simulink model "simulacao_manipulador_scara_Anne"  (R2022b)
settings: Solver=ode1  StartTime=0.0  StopTime=20  FixedStep=1e-4  RelTol=1e-3
values from neighbouring files (symbols this model uses):
  L1_num = 0.525    [testeSCARA.m]
  L2_num = 0.330    (= 0.33)    [testeSCARA.m]
  Lf_num = 0.07673    [testeSCARA.m]
undefined symbols (not defined in the file or in its folder): deltat, dq_ci, Kd, Kp, L0_num, PA_0, PB_0, PD_0, q_ci, Tpi_0, trajetLin1
settings Model: Creator=alefp  LastModifiedBy=rodrigo
settings OptimizationCC: DefaultParameterBehavior=Inlined  ReuseModelBlockBuffer=on  EnhancedBackFolding=on  PassReuseOutputArgsThreshold=0  OptimizeBlockOrder=speed  DifferentSizesBufferReuse=on  OptimizationCustomize=off
settings DebuggingCC: ReadBeforeWriteMsg=DisableAll  WriteAfterWriteMsg=DisableAll  WriteAfterReadMsg=DisableAll  MultiTaskDSMMsg=none  ParameterTunabilityLossMsg=error
settings ModelReferenceCC: UpdateModelReferenceTargets=IfOutOfDate
settings SFSimCC: SFSimEcho=off  MATLABDynamicMemAlloc=off
settings CodeAppCC: ForceParamTrailComments=on  OperatorAnnotations=on

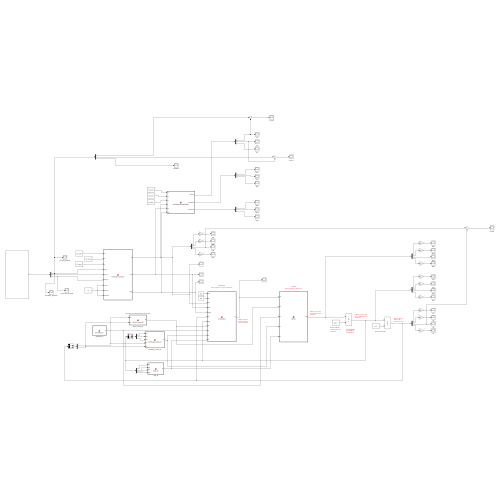
[thumbnail: Simulink's stored preview of the top-level diagram]
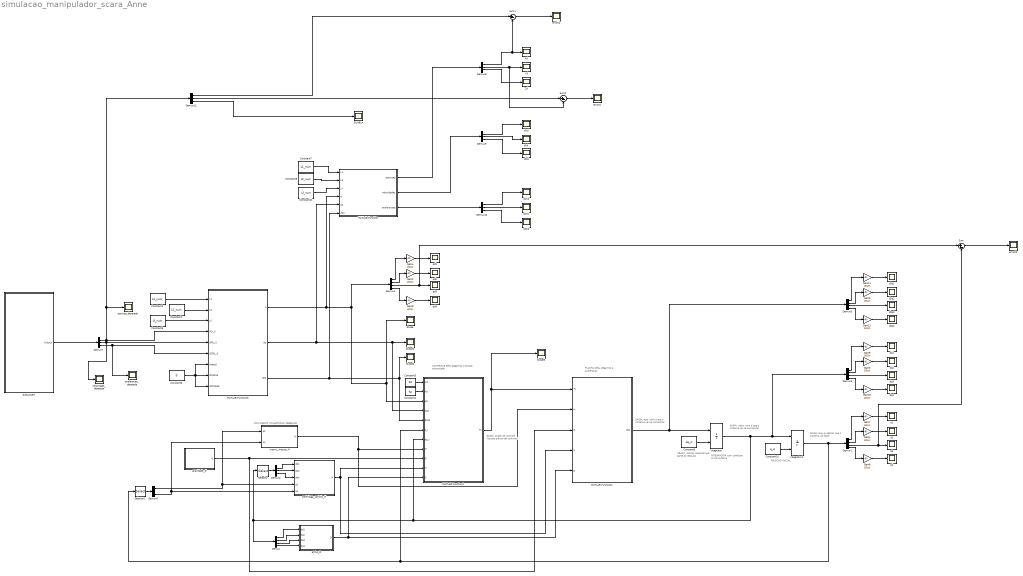
== system simulacao_manipulador_scara_Anne ==
  note: MOVIMENTO (TRAJETÓRIA) DESEJADO
  note: CONTROLE
      | Dele, pegamos o torque computado
  note: PLANTA
      | Dela, pegamos a aceleracao
  note: INTEGRADOR
      | com condicao inicial externa
  note: VELOC. INICIAL
      | Supondo que parte do repouso
  note: POSICAO INICIAL
  note: SAIDA: ang. ou desloc que o sistema vai fazer
  note: SAIDA: veloc. com a que o sistema vai se comportar
  note: SAIDA: acel. com a que o sistema vai se comportar
  note: SAIDA: acoes de controle (torque e forca de controle)
  BLABLA : Scope
  Constant1 : Constant  Value=L1_num
  Constant10 : Constant  Value=q_ci
  Constant11 : Constant  Value=Lf_num
  Constant2 : Constant  Value=L2_num
  Constant3 : Constant  Value=Kd
  Constant4 : Constant  Value=Kp
  Constant5 : Constant  Value=Lf_num
  Constant6 : Constant  Value=0
  Constant7 : Constant  Value=L1_num
  Constant8 : Constant  Value=L2_num
  Constant9 : Constant  Value=dq_ci
  Demux{,1,3..5} (5 alike) : Demux
  Demux{2,7..11} (6 alike) : Demux  Outputs=3
  Demux6 : Demux  Outputs=2
  Gain{1..12} (12 alike) : Gain  Gain=180/pi
  Integrator : Integrator  InitialConditionSource=external
  Integrator1 : Integrator  InitialConditionSource=external
  MATLAB Function : MATLAB Function  TreatAsAtomicUnit=on
  MATLAB Function1 : MATLAB Function  TreatAsAtomicUnit=on
  MATLAB Function2 : MATLAB Function  TreatAsAtomicUnit=on
  MATLAB Function3 : MATLAB Function  TreatAsAtomicUnit=on
  Scope{,1..3} (4 alike) : Scope
  Selector : Selector  InputPortWidth=4  IndexOptions=Index vector (dialog)  Indices=[1, 2, 4]  OutputSizes=1
  Selector1 : Selector  InputPortWidth=4  IndexOptions=Index vector (dialog)  Indices=[2, 4]  OutputSizes=1
  Subsystem : Subsystem
  Sum : Sum  Inputs=|+-
  Sum1 : Sum  Inputs=|+-
  Sum2 : Sum  Inputs=|+-
  Xd : Scope
  Yd : Scope
  Zd : Scope
  aceleracao_desejada : Scope
  atrito_D : MATLAB Function  TreatAsAtomicUnit=on
  centrifuga_coriolis_H : MATLAB Function  TreatAsAtomicUnit=on
  d2Xd : Scope
  d2Yd : Scope
  d2Zd : Scope
  d2q{1..4} (4 alike) : Scope
  dXd : Scope
  dYd : Scope
  dZd : Scope
  dq{1..4} (4 alike) : Scope
  erroQ3 : Scope
  erroXd : Scope
  erroYd : Scope
  gravidade_G : MATLAB Function  TreatAsAtomicUnit=on
  matriz_massa_M : MATLAB Function  TreatAsAtomicUnit=on
  posicao_desejada : Scope
  q{1..4} (4 alike) : Scope
  qd{1..4} (4 alike) : Scope
  velocidade_desejada : Scope
  wires:
  MATLAB Function3/2(dq) -> MATLAB Function/5(dq), MATLAB Function1/4(dqd), Scope1/1
  MATLAB Function3/3(d2q) -> MATLAB Function/6(d2q), MATLAB Function1/5(d2qd), Scope2/1
  MATLAB Function3/1(q) -> MATLAB Function/4(q), Scope/1, MATLAB Function1/3(qd), Demux4/1
  MATLAB Function1/1(Tc) -> Scope3/1, MATLAB Function2/1(Tc)
  Constant9/1 -> Integrator/2
  Constant10/1 -> Integrator1/2
  Demux4/1 -> Gain4/1
  Gain4/1 -> qd1/1
  matriz_massa_M/1(M) -> MATLAB Function2/2(M), MATLAB Function1/8(M)
  gravidade_G/1(G) -> MATLAB Function2/3(G), MATLAB Function1/9(G)
  centrifuga_coriolis_H/1(H) -> MATLAB Function1/10(H), MATLAB Function2/4(H)
  atrito_D/1(D) -> MATLAB Function1/11(D), MATLAB Function2/5(D)
  Gain2/1 -> qd2/1
  Demux4/2 -> Gain2/1
  Gain6/1 -> qd4/1
  Demux4/4 -> Gain6/1
  Demux/1 -> atrito_D/1(dq1)
  Demux/2 -> atrito_D/2(dq2)
  Demux/3 -> atrito_D/3(dq3)
  Demux/4 -> atrito_D/4(dq4)
  Demux2/2 -> centrifuga_coriolis_H/2(dq2)
  Demux2/1 -> centrifuga_coriolis_H/1(dq1)
  Selector/1 -> Demux2/1
  Demux6/1 -> matriz_massa_M/1(q2), centrifuga_coriolis_H/4(q2)
  Selector1/1 -> Demux6/1
  Demux1/4 -> Gain8/1
  Demux1/3 -> Sum/2, q3/1
  Demux1/1 -> Gain7/1
  Demux1/2 -> Gain1/1
  Integrator1/1 -> MATLAB Function1/6(q_r), Selector1/1, Demux1/1
  Gain1/1 -> q2/1
  Gain8/1 -> q4/1
  Gain7/1 -> q1/1
  Demux3/4 -> Gain10/1
  Demux3/3 -> dq3/1
  Demux3/1 -> Gain9/1
  Demux3/2 -> Gain3/1
  Integrator/1 -> Demux3/1, Integrator1/1, Selector/1, Demux/1, MATLAB Function1/7(dq_r)
  Gain3/1 -> dq2/1
  Gain10/1 -> dq4/1
  Gain9/1 -> dq1/1
  Demux5/4 -> Gain12/1
  Demux5/3 -> d2q3/1
  Demux5/1 -> Gain11/1
  Demux5/2 -> Gain5/1
  MATLAB Function2/1(d2q) -> Demux5/1, Integrator/1
  Gain5/1 -> d2q2/1
  Gain12/1 -> d2q4/1
  Gain11/1 -> d2q1/1
  Constant3/1 -> MATLAB Function1/1(Kd)
  Constant4/1 -> MATLAB Function1/2(Kp)
  Demux6/2 -> centrifuga_coriolis_H/5(q4), matriz_massa_M/2(q4)
  Constant1/1 -> MATLAB Function3/1(L1)
  Constant2/1 -> MATLAB Function3/2(L2)
  Constant5/1 -> MATLAB Function3/3(Lf)
  Constant6/1 -> MATLAB Function3/9(d2theta5), MATLAB Function3/7(theta5), MATLAB Function3/8(dtheta5)
  Demux7/2 -> velocidade_desejada/1, MATLAB Function3/5(dPQ_0)
  Demux7/3 -> MATLAB Function3/6(d2PQ_0), aceleracao_desejada/1
  Demux7/1 -> Demux11/1, posicao_desejada/1, MATLAB Function3/4(PQ_0)
  Subsystem/1(Output) -> Demux7/1
  Demux2/3 -> centrifuga_coriolis_H/3(dq4)
  Sum/1 -> erroQ3/1
  Constant7/1 -> MATLAB Function/1(L1)
  Constant8/1 -> MATLAB Function/2(L2)
  Constant11/1 -> MATLAB Function/3(Lf)
  Sum1/1 -> erroXd/1
  Demux4/3 -> Sum/1, qd3/1
  MATLAB Function/3(aceleracoes) -> Demux10/1
  MATLAB Function/2(velocidades) -> Demux9/1
  MATLAB Function/1(posicoes) -> Demux8/1
  Demux8/3 -> Zd/1
  Demux8/2 -> Sum2/2, Yd/1
  Demux8/1 -> Sum1/2, Xd/1
  Demux9/3 -> dZd/1
  Demux9/2 -> dYd/1
  Demux9/1 -> dXd/1
  Demux10/3 -> d2Zd/1
  Demux10/2 -> d2Yd/1
  Demux10/1 -> d2Xd/1
  Demux11/1 -> Sum1/1
  Demux11/2 -> Sum2/1
  Sum2/1 -> erroYd/1
  Demux11/3 -> BLABLA/1

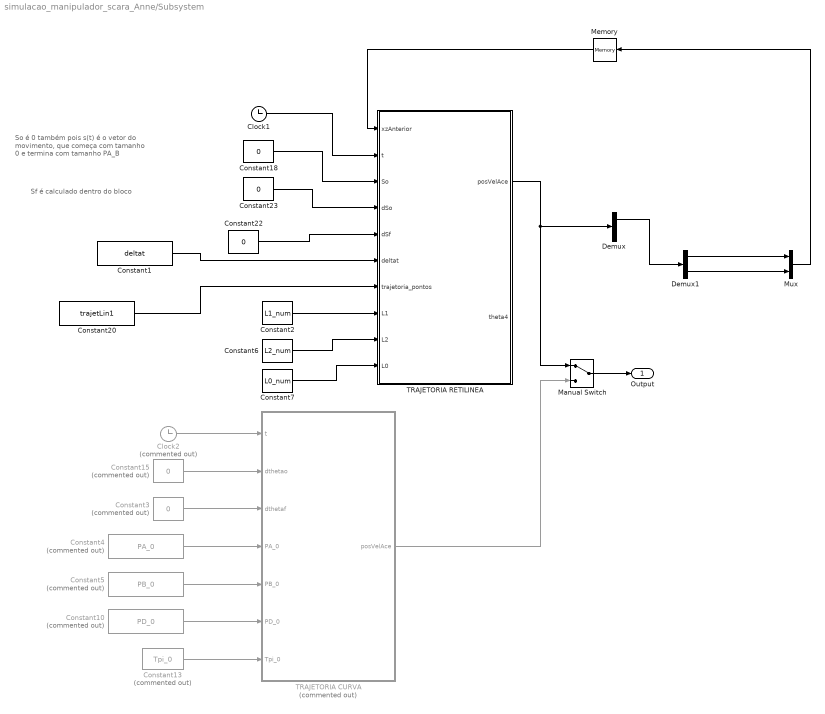
== system simulacao_manipulador_scara_Anne/Subsystem ==
  note: Sf é calculado dentro do bloco
  note: So é 0 também pois s(t) é o vetor do movimento, que começa com tamanho 0 e termina com tamanho PA_B
  Clock1 : Clock
  Clock2 : Clock  Commented=on
  Constant1 : Constant  Value=deltat
  Constant10 : Constant  Commented=on  Value=PD_0
  Constant13 : Constant  Commented=on  Value=Tpi_0
  Constant15 : Constant  Commented=on  Value=0
  Constant18 : Constant  Value=0
  Constant2 : Constant  Value=L1_num
  Constant20 : Constant  Value=trajetLin1
  Constant22 : Constant  Value=0
  Constant23 : Constant  Value=0
  Constant3 : Constant  Commented=on  Value=0
  Constant4 : Constant  Commented=on  Value=PA_0
  Constant5 : Constant  Commented=on  Value=PB_0
  Constant6 : Constant  Value=L2_num
  Constant7 : Constant  Value=L0_num
  Demux : Demux  Outputs=3
  Demux1 : Demux  Outputs=3
  Manual Switch : ManualSwitch
  Memory : Memory
  Mux : Mux  Inputs=2
  TRAJETORIA CURVA : MATLAB Function  Commented=on  TreatAsAtomicUnit=on
  TRAJETORIA RETILINEA : MATLAB Function  TreatAsAtomicUnit=on
  Output : Outport
  wires:
  Constant4/1 -> TRAJETORIA CURVA/4(PA_0)
  Constant3/1 -> TRAJETORIA CURVA/3(dthetaf)
  Clock2/1 -> TRAJETORIA CURVA/1(t)
  Constant15/1 -> TRAJETORIA CURVA/2(dthetao)
  Constant5/1 -> TRAJETORIA CURVA/5(PB_0)
  Constant10/1 -> TRAJETORIA CURVA/6(PD_0)
  Manual Switch/1 -> Output/1
  TRAJETORIA CURVA/1(posVelAce) -> Manual Switch/2
  Constant13/1 -> TRAJETORIA CURVA/7(Tpi_0)
  Constant22/1 -> TRAJETORIA RETILINEA/5(dSf)
  Clock1/1 -> TRAJETORIA RETILINEA/2(t)
  Constant18/1 -> TRAJETORIA RETILINEA/3(So)
  Constant23/1 -> TRAJETORIA RETILINEA/4(dSo)
  Constant1/1 -> TRAJETORIA RETILINEA/6(deltat)
  TRAJETORIA RETILINEA/1(posVelAce) -> Demux/1, Manual Switch/1
  Mux/1 -> Memory/1
  Memory/1 -> TRAJETORIA RETILINEA/1(xzAnterior)
  Demux/1 -> Demux1/1
  Demux1/1 -> Mux/1
  Demux1/3 -> Mux/2
  Constant20/1 -> TRAJETORIA RETILINEA/7(trajetoria_pontos)
  Constant2/1 -> TRAJETORIA RETILINEA/8(L1)
  Constant6/1 -> TRAJETORIA RETILINEA/9(L2)
  Constant7/1 -> TRAJETORIA RETILINEA/10(L0)

== matlab function simulacao_manipulador_scara_Anne/atrito_D ==
  data: dq1 input; D output; dq2 input; dq3 input; dq4 input
function D = atrito_D(dq1,dq2,dq3,dq4)
%#codegen

%    This function was generated by the Symbolic Math Toolbox version 24.2.
%    25-Sep-2024 18:08:51

% dq1 = complex(dq1);  % if required to enforce complex operations
% dq2 = complex(dq2);  % if required to enforce complex operations
% dq3 = complex(dq3);  % if required to enforce complex operations
% dq4 = complex(dq4);  % if required to enforce complex operations
D = [dq1.*9.321584999999999e-3;dq2.*2.192184e-2;dq3.*1.74398e-4;dq4.*2.754e-4];
end

== matlab function simulacao_manipulador_scara_Anne/MATLAB Function3 ==
  data: L1 input; L2 input; q output; Lf input; PQ_0 input; dPQ_0 input; d2PQ_0 input; theta5 input; dq output; d2q output; dtheta5 input; d2theta5 input
function [q, dq, d2q]  = cinematica_inversa(L1, L2, Lf, PQ_0,dPQ_0, d2PQ_0, theta5, dtheta5, d2theta5)
    % theta5 é o angulo final da ferramenta, conseguido pela tarefa. Lembrando que q4 = theta5 - q1 - q2 
    % PQ_0: Vetor de posicoes desejadas
    % dPQ_0: Vetor de velocidades desejadas (linear e angular)
    % d2PQ_0: Vetor de acelerações desejadas
    
    x5 = PQ_0(1);
    y5 = PQ_0(2);
    z5 = PQ_0(3);
    
    %% Cálculo de q3 (componente prismática)
    % q3 é o deslocamento da junta prismática
    q3 = y5 + Lf;
    
    num = (x5^2 + z5^2 - L1^2 - L2^2);
    den = (2*L1*L2);

    % Truncando na 3ª casa decimal
    num = fix(num * 1000) / 1000;
    den = fix(den * 1000) / 1000;
    q2 = acos(num/den);
    if sao_valores_proximos(q2,0) || sao_valores_proximos(q2,pi) || sao_valores_proximos(q2,2*pi)
        q2 =+ 0.087; % acrescentando 5 graus
    end
    

    %% Cálculo de q1 (componente rotacional)
    q1 = atan2(-L2*sin(q2)*x5 - (L1 + L2*cos(q2))*z5, (L1 + L2*cos(q2))*x5 - L2*sin(q2)*z5);

    %% Cálculo de q4 (componente rotacional)
    q4 = theta5 - q1 - q2;
    
    %% Atribuiçao das variáveis de saida - posicao e angulos
    q = [q1; q2; q3; q4];

    %% Calculo das velocidades - derivada primeira - angulares e lineares

    % Jacobiano completo (linhas para velocidades lineares e angulares)
    % Colocamos as derivadas parciais de x5, y5, z5 e theta5 em relação às variáveis articulares
    J = [
        - L2 * sin(q1 + q2) - L1 * sin(q1), - L2 * sin(q1 + q2), 0, 0;  % dx/dq1, dx/dq2, dx/dq3, dx/dq4
        0, 0, 1, 0; % dy/dq1, dy/dq2, dy/dq3, dy/dq4
        - L2 * cos(q1 + q2) - L1 * cos(q1), - L2 * cos(q1 + q2), 0, 0; % dz/dq1, dz/dq2, dz/dq3, dz/dq4
        1, 1, 0, 1 % dtheta5/dq1, dtheta5/dq2, dtheta5/dq3, dtheta5/dq4
    ];

    
    dPQ_0 = [dPQ_0; dtheta5];

    % Resolvendo para as velocidades articulares
    dq = J \ dPQ_0; % Usando \ para maior precisão em vez de inv(J)

    %% Calculo das aceleracoes - derivada segunda - angulares e lineares
    dq1 = dq(1);
    dq2 = dq(2);
    % Derivada do Jacobiano
    dJ = [
        -L2*cos(q1 + q2)*(dq1 + dq2) - L1*cos(q1)*dq1,  -L2*cos(q1 + q2)*(dq1 + dq2),  0,  0;
        0, 0, 0, 0;
        L2*sin(q1 + q2)*(dq1 + dq2) + L1*sin(q1)*dq1,   L2*sin(q1 + q2)*(dq1 + dq2),  0,  0;
        0, 0, 0, 0
    ];    
    % Vetor de acelerações desejadas
    d2PQ_0 = [d2PQ_0; d2theta5];  % Aceleração linear e angular desejadas
    
    % Calculando a aceleração inversa
    d2q = J \ (d2PQ_0 - dJ * dq);  % Usando \ (backslash) em vez de inv(J) para maior precisão

end

== matlab function simulacao_manipulador_scara_Anne/Subsystem/TRAJETORIA CURVA ==
  data: t input; dthetao input; dthetaf input; PA_0 input; PB_0 input; PD_0 input; posVelAce output; Tpi_0 input
function posVelAce = posVelAce(t, dthetao, dthetaf, PA_0, PB_0, PD_0, Tpi_0)

% Itens marcados com '*' dever ser fornecidos pelo usuario 

% Parâmetros de entrada:
% t          - tempo atual da simulação
% dthetao    - velocidade angular inicial
% dthetaf    - velocidade angular final
% deltat     - tempo total da trajetória (em segundos)
% PA_0       - coordenadas do ponto A
% PB_0       - coordenadas do ponto B
% PD_0       - coordenadas do ponto D (terceiro ponto)
% L1, L2     - tamanhos das partes do manipulador

% Definindo limites para a área de controle
%raio_min = L1;           % Raio mínimo com a junta prismática retraída
%raio_max = L1 + L2;      % Raio máximo com a junta prismática estendida



% Definindo os intervalos de tempo
if t >= 0 && t <= 10
    %% Fase 1: Tempo de 0 a 9 segundos
    to = 0;
    tf = 10;  % Duração do intervalo (10 segundos)

    %~~~~~~~~~~~~~~ AUXILIAR PARA EXEMPLO SCARA 4GDLs ~~~~~~~~~~~~~~~~~~
    % Achando os pontos A, B e D na base {pi}
    PA_pi = Tpi_0^-1*[PA_0; 1];
    PB_pi = Tpi_0^-1*[PB_0; 1];
    PD_pi = Tpi_0^-1*[PD_0; 1];
    
    % Reduzindo os pontos para as duas dimensoes do plano pi
    PA_pi = PA_pi(1:2);
    PB_pi = PB_pi(1:2);
    PD_pi = PD_pi(1:2);


    %~~~~~~~~~~~~~~~~~~~~~~~~~~~~~~~~~~~~~~~~~~~~~~~~~~~~~~~~~~~~~~~~~~~
    

    % Calculando o centro da circunferência (C) a partir dos três pontos A, B, e D
    [C, R] = calcularCentroCircunferencia(PA_pi, PB_pi, PD_pi);

    % Vetores CA e CB
    CA = PA_pi - C;
    CB = PB_pi - C;
    
    % Ângulo inicial (em relação ao ponto C)
    thetao = atan2(CA(2), CA(1));  % Ângulo em radianos
    %thetao = rad2deg(thetao)
    
    % Ângulo final (em relação ao ponto C)
    thetaf = atan2(CB(2), CB(1));  % Ângulo em radianos
    %thetaf = rad2deg(thetaf)
    
    % Ajustar ângulos para o intervalo [0, 2*pi] (em radianos)
    if thetao < 0
        thetao = thetao + 2*pi;
    end
    
    if thetaf < 0
        thetaf = thetaf + 2*pi;
    end
else
    % Se t não está nos intervalos esperados, atribuir valores padrão
    to = 0;
    tf = 0;
    PQ_0 = [0; 0; 0];
    dPQ_0 = [0; 0; 0];
    d2PQ_0 = [0; 0; 0];
    posVelAce = [PQ_0; dPQ_0; d2PQ_0];
    % posVelAce = PQ_0;
    return;
end

%% Trajetória cúbica para theta(t), dtheta(t), e d2theta(t)
% Coeficientes da equação cúbica para interpolação angular
A = [1 to to^2 to^3; 0 1 2*to 3*to^2; 1 tf tf^2 tf^3; 0 1 2*tf 3*tf^2];
b = [thetao; dthetao; thetaf; dthetaf];
a = inv(A)*b; % Coeficientes cúbicos [a0; a1; a2; a3]

% Calculando o ângulo (theta), velocidade angular (dtheta) e aceleração angular (d2theta)
thetat = a(1) + a(2)*t + a(3)*t^2 + a(4)*t^3;
dthetat = a(2) + 2*a(3)*t + 3*a(4)*t^2;
d2thetat = 2*a(3) + 6*a(4)*t;

%% Calculando a posição, velocidade e aceleração ao longo da curva
% Raio da circunferência já foi calculado como R a partir de A, B, D

% Posição ao longo do arco de círculo
PQ_pi = [C(1) + R * cos(thetat);   % Coordenada X do ponto no arco
        C(2) + R * sin(thetat)];  % Coordenada Y do ponto no arco


PQ_0 = Tpi_0*[PQ_pi; 0; 1];
PQ_0 = PQ_0(1:3);


% Cálculo da distância do ponto G à origem (0,0)
distancia_G = sqrt(PQ_0(1)^2 + PQ_0(2)^2 + + PQ_0(3)^2);

% Vetor tangente (normalizado) à curva circular em cada ponto
tangente = [-sin(thetat), cos(thetat)]; % Vetor tangente é perpendicular ao vetor radial
tangente = tangente / norm(tangente);   % Normalizando o vetor tangente

% Velocidade ao longo do arco (direção tangente)
dPQ_0 = dthetat * R * tangente'; % Multiplicando pela velocidade angular e o raio
dPQ_0 = Tpi_0*[dPQ_0; 0; 1];
dPQ_0 = dPQ_0(1:3);

% Aceleração ao longo do arco (direção tangente)
d2PQ_0 = d2thetat * R * tangente'; % Multiplicando pela aceleração angular e o raio
d2PQ_0 = Tpi_0*[d2PQ_0; 0; 1];
d2PQ_0 = d2PQ_0(1:3);

% ================= VERIFICAR SE PQ_0 ESTA DENTRO DA AREA DE CONTROLE ====================
% % Verificando se a distância está fora dos limites
% if distancia_G < raio_min || distancia_G > raio_max
%     disp('Atenção: A trajetória sai da área de controle! Simulação não pode ser executada.');
%     posVelAce = [PQ_0; dPQ_0; d2PQ_0];
%     return;
% end
% ========================================================================================

%% Resultado final
% Retornar a posição, velocidade e aceleração como uma matriz 6x1

posVelAce = [PQ_0; dPQ_0; d2PQ_0];
% posVelAce = PQ_0;

end

%% Função auxiliar para calcular o centro do círculo
function [C, R] = calcularCentroCircunferencia(A, B, D)

    % Coordenadas dos pontos A, B, e D
    xA = A(1); yA = A(2);
    xB = B(1); yB = B(2);
    xD = D(1); yD = D(2);
    
    % Subtraímos as equações para eliminar R^2
    % Subtraindo equacao_B de equacao_A:
    F1 = (xB^2 + yB^2) - (xA^2 + yA^2);
    G1 = 2 * (xB - xA);
    H1 = 2 * (yB - yA);
    
    % Subtraindo equacao_D de equacao_A:
    F2 = (xD^2 + yD^2) - (xA^2 + yA^2);
    G2 = 2 * (xD - xA);
    H2 = 2 * (yD - yA);
    
    % Sistema de equações linear para xC e yC:
    A_eq = [G1, H1; G2, H2];
    b_eq = [F1; F2];
    
    % Resolvendo o sistema linear
    C = A_eq \ b_eq; % C = inv(A_eq)*b_eq
    
    % Centro da circunferência
    xC = C(1);
    yC = C(2);
    
    % Calculando o raio da circunferência (usando o ponto A para calcular R)
    R = sqrt((xA - xC)^2 + (yA - yC)^2);

end

== matlab function simulacao_manipulador_scara_Anne/Subsystem/TRAJETORIA RETILINEA ==
  data: xzAnterior input; t input; So input; posVelAce output; dSo input; dSf input; deltat input; theta4 output; trajetoria_pontos input; L1 input; L2 input; L0 input
function [posVelAce, theta4]  = posVelAce( xzAnterior, t, So, dSo, dSf, deltat, trajetoria_pontos,L1,L2,L0)
    
    
    % Parâmetros de entrada:
    % xzAnterior - Coordenadas x e z da iteração anterior
    % trajetoria_pontos - Posições das trajetórias definidas para o manipulador 
    % t          - tempo atual da simulação
    % So, Sf     - posições inicial e final
    % dSo, dSf   - velocidades iniciais e finais
    % deltat     - tempo total da trajetória (em segundos)
    % PA_0       - coordenadas do ponto A
    % PB_0       - coordenadas do ponto B
    % L1, L2     - Comprimentos das partes do manipulador
    
    % Definindo limites para a área de controle
    % raio_min = L1;           % Raio mínimo com a junta prismática retraída
    % raio_max = L1 + L2;      % Raio máximo com a junta prismática estendida
    
    % SELEÇÃO DE TRAJETÓRIA

    % MOVIMENTO 1
    if t <= deltat(1)
        to = 0;
        tf = deltat(1); % Duração total do movimento
        % dSo = .05;
        % d2So = -.005
        % 
        % dSf = .05;
        % d2Sf = .005
        PA_0 = trajetoria_pontos(1:3);
        PB_0 = trajetoria_pontos(4:6);
        posVelAce = calcular_trajetoria3(PA_0, PB_0, t, So, dSo, dSf,  to, tf);
        % posVelAce = calcular_trajetoria5(PA_0, PB_0, t, So, dSo, d2So, dSf, d2Sf, to, tf);
        theta4 = calcular_orientacao(posVelAce(1:3))
   
    % MOVIMENTO 2
    elseif t >= deltat(1) && t <= (deltat(1) + deltat(2)) % MOVIMENTO 2
        % Atualizando o ponto de partida (usando PB_0 da fase anterior)
        PA_0 = trajetoria_pontos(7:9);
        PB_0 = trajetoria_pontos(10:12);
        to = deltat(1);
        tf = deltat(1) + deltat(2); % Duração total do movimento

        % dSo = .05;
        % d2So = -.005
        % 
        % dSf = .05;
        % d2Sf = .005

        posVelAce = calcular_trajetoria3(PA_0, PB_0, t, So, dSo, dSf,  to, tf);
        % posVelAce = calcular_trajetoria5(PA_0, PB_0, t, So, dSo, d2So, dSf, d2Sf, to, tf);
        theta4 = calcular_orientacao(posVelAce(1:3))

    % MOVIMENTO 3
    % elseif t >= (deltat(1) + deltat(2)) && t <= (deltat(1) + deltat(2) + deltat(3))
    %     PA_0 = trajetoria_pontos(13:15);
    %     PB_0 = trajetoria_pontos(16:18);
    %     to = deltat(1) + deltat(2);
    %     tf = deltat(1) + deltat(2) + deltat(3); % Duração total do movimento
    %     posVelAce = calcular_trajetoria3(PA_0, PB_0, t, So, dSo, dSf,  to, tf);
    %     theta4 = calcular_orientacao(posVelAce(1:3))

    % MOVIMENTO 4
    % elseif t >= (deltat(1) + deltat(2) + deltat(3)) && t <= (deltat(1) + deltat(2) + deltat(3) + deltat(4))
    %     PA_0 = trajetoria_pontos(19:21);
    %     PB_0 = trajetoria_pontos(22:24);
    %     to = deltat(1) + deltat(2) + deltat(3);
    %     tf = deltat(1) + deltat(2) + deltat(3) + deltat(4); % Duração total do movimento
    %     posVelAce = calcular_trajetoria3(PA_0, PB_0, t, So, dSo, dSf,  to, tf);
    %     theta4 = calcular_orientacao(posVelAce(1:3))


    else
        % Se t está fora do intervalo esperado, atribuir valores padrão
        PQ_0 = [0; 0; 0];
        dPQ_0 = [0; 0; 0];
        d2PQ_0 = [0; 0; 0];
        posVelAce = [PQ_0; dPQ_0; d2PQ_0];
        theta4 = 0;
    end



    function [theta4] = calcular_orientacao(posVelAce)

        % Calcula a tangente da trajetória
        PQ_0 = posVelAce;  % Posição atual [x, y, z]
        xzAtual = [PQ_0(1); PQ_0(3)];  % Extrai x e z atuais
    
        % Cálculo da tangente (diferença entre as coordenadas atuais e anteriores)
        tangente = xzAtual - xzAnterior;
        
        % Normalizando o vetor tangente (vetor unitario na direcao tanjente à trajetoria) 
        tangente_normalizado = tangente / norm(tangente)
    
        % Atualizar xzAnterior com os valores atuais para a próxima iteração (realimentação)
        %xzAnterior = xzAtual;  % Isso deve ser armazenado para a próxima iteração
    
        % A tangente é usada para calcular o ângulo theta4
        theta4 = atan2(tangente_normalizado(2), tangente_normalizado(1));
        
        % Matriz de rotação R_4_0 baseada em theta4
        R_4_0 = [cos(theta4), 0, sin(theta4);
                 0, 1, 0;
                -sin(theta4), 0, cos(theta4)]
    
        theta4 = rad2deg(atan2(R_4_0(1,3), R_4_0(3,3)));
    end






    
    % Função auxiliar para calcular a trajetória cúbica
    function [posVelAce] = calcular_trajetoria3(PA_0, PB_0, t, So, dSo, dSf, to, tf)
        %% CALCULO VETOR UNITARIO
        % Calculando o vetor de A para B
        AB_vector = PB_0 - PA_0;
        
        % Calculando o vetor unitário de A para B
        unitAB_0 = AB_vector / norm(AB_vector);
        
        % Calculando o vetor de A para B (PA_B)
        PA_B = PB_0 - PA_0;
        
        % Calculando o módulo (norma) do vetor PA_B
        modulo_PA_B = norm(PA_B);
        Sf = modulo_PA_B; % tamanho final do vetor s
        
        %% POSICAO, VELOCIDADE e ACELERACAO
        % Definindo os coeficientes para a trajetória cúbica
        A = [1 to to^2 to^3; 0 1 2*to 3*to^2; 1 tf tf^2 tf^3; 0 1 2*tf 3*tf^2];
        b = [So; dSo; Sf; dSf];
        a = A \ b; % Coeficientes cúbicos [a0; a1; a2; a3]
        
        % Calculando a posição, velocidade e aceleração ao longo do tempo
        st = a(1) + a(2)*t + a(3)*t^2 + a(4)*t^3; % este s é o percurso
        dst = a(2) + 2*a(3)*t + 3*a(4)*t^2;       % Velocidade ao longo da trajetória
        d2st = 2*a(3) + 6*a(4)*t;                 % Aceleração ao longo da trajetória
    
        %% CALCULO POSICAO, ACELERACAO e VELOCIDADE EM RELACAO AO INCERCIAL 
        PQ_0 = st*unitAB_0 + PA_0;  % Somando a posição inicial
        dPQ_0 = dst*unitAB_0;       % Velocidade
        d2PQ_0 = d2st*unitAB_0;     % Aceleração
    
        xf = PQ_0(1);
        yf = PQ_0(2);
        zf = PQ_0(3);
        if areaDeTrabalhoInvalida(xf,yf,zf,L1,L2,L0)
            error('O ponto {xf=%d}, {yf=%d}, {zf=%d} esta fora da area de trabalho!',xf,yf,zf)
        end
        %% Saída: posição, velocidade e aceleração
        posVelAce = [PQ_0; dPQ_0; d2PQ_0];
    end





    % Função auxiliar para calcular a trajetória cúbica
    function [posVelAce] = calcular_trajetoria5(PA_0, PB_0, t, So, dSo, d2So, dSf, d2Sf, to, tf)
        %% CALCULO VETOR UNITARIO
        % Calculando o vetor de A para B
        AB_vector = PB_0 - PA_0;
        
        % Calculando o vetor unitário de A para B
        unitAB_0 = AB_vector / norm(AB_vector);
        
        % Calculando o vetor de A para B (PA_B)
        PA_B = PB_0 - PA_0;
        
        % Calculando o módulo (norma) do vetor PA_B
        modulo_PA_B = norm(PA_B);
        Sf = modulo_PA_B; % tamanho final do vetor s
        
        %% POSICAO, VELOCIDADE e ACELERACAO
        % Definindo os coeficientes para a trajetória cúbica
        A = [1 to to^2 to^3 to^4 to^5;  
            0 1 2*to 3*to^2 4*to^3 5*to^4;
            0 0 2 6*to 12*to^2 20*to^3;
            1 tf tf^2 tf^3 tf^4 tf^5;  
            0 1 2*tf 3*tf^2 4*tf^3 5*tf^4;
            0 0 2 6*tf 12*tf^2 20*tf^3];
        b = [So; dSo; d2So; Sf; dSf; d2Sf];
        a = A \ b; % Coeficientes cúbicos [a0; a1; a2; a3]
        
        % Calculando a posição, velocidade e aceleração ao longo do tempo

        st = a(1) + a(2)*t + a(3)*t^2 + a(4)*t^3 + a(5)*t^4 + a(6)*t^5  % este s é o percurso
        dst = a(2) + 2*a(3)*t + 3*a(4)*t^2 + 4*a(5)*t^3 + 5*a(6)*t^4    % Velocidade ao longo da trajetória
        d2st = 2*a(3) + 6*a(4)*t + 12*a(5)*t^2 + 20*a(6)*t^3            % Aceleração ao longo da trajetória

        %% CALCULO POSICAO, ACELERACAO e VELOCIDADE EM RELACAO AO INCERCIAL 
        PQ_0 = st*unitAB_0 + PA_0;  % Somando a posição inicial
        dPQ_0 = dst*unitAB_0;       % Velocidade
        d2PQ_0 = d2st*unitAB_0;     % Aceleração
        if areaDeTrabalhoInvalida(xf,yf,zf,L1,L2,L0)
            error('O ponto {x=%d}, {y=%d}, {z=%d} esta fora da area de trabalho!')
        end
        %% Saída: posição, velocidade e aceleração
        posVelAce = [PQ_0; dPQ_0; d2PQ_0];
    end
end

== matlab function simulacao_manipulador_scara_Anne/MATLAB Function1 ==
  data: Kd input; Kp input; Tc output; qd input; dqd input; d2qd input; q_r input; dq_r input; M input; G input; H input; D input
function Tc  = controlador(Kd, Kp, qd, dqd, d2qd, q_r, dq_r, M, G, H, D)
Tc = M*(d2qd + Kd*(dqd-dq_r) + Kp*(qd- q_r)) + H + G + D;

== matlab function simulacao_manipulador_scara_Anne/MATLAB Function ==
  data: L1 input; posicoes output; velocidades output; L2 input; Lf input; q input; dq input; d2q input; aceleracoes output
function [posicoes, velocidades, aceleracoes] = cinematicaDiretaSCARA(L1, L2, Lf, q, dq, d2q)
    % DIRETA_SCARA .......
    % RRPR

    P_1 = [L1; 0; 0];
    P_2 = [L2; 0; 0];
    P_3 = [0; q(3); 0];
    P_5 = [0; Lf; 0]; % ferramenta

    q1 = q(1);
    q2 = q(2); 
    q3 = q(3);
    q4 = q(4);

    dq1 = dq(1);
    dq2 = dq(2); 
    dq3 = dq(3);
    dq4 = dq(4);

    d2q1 = d2q(1);
    d2q2 = d2q(2); 
    d2q3 = d2q(3);
    d2q4 = d2q(4);

    %% Elo 1:
    R_y_q1 = RotacaoPura('y',q1);
    D_1_0_P1 = TranslacaoPura(P_1);
    transformacoesPuras_1_0 = {R_y_q1,D_1_0_P1};
    [col_Ja_1,T_1_0] = transformacoesCombinadas(eye(4),transformacoesPuras_1_0);
    P_1_0 = T_1_0(1:3, 4);

    %% Elo 2:
    R_y_q2 = RotacaoPura('y',q2);
    D_2_1_P2 = TranslacaoPura(P_2);
    transformacoesPuras_2_1 = {R_y_q2,D_2_1_P2};
    [col_Ja_2, T_2_0] = transformacoesCombinadas(T_1_0,transformacoesPuras_2_1);
    P_2_0 = T_2_0(1:3, 4);

    %% Elo 3:
    D_3_2_P3 = TranslacaoPura(P_3);
    transformacoesPuras_3_2 = {D_3_2_P3};
    [col_Ja_3, T_3_0] = transformacoesCombinadas(T_2_0,transformacoesPuras_3_2);
    P_3_0 = T_3_0(1:3, 4);

    %% Elo 4:
    R_y_q4 = RotacaoPura('y',q4);
    transformacoesPuras_4_3 = {R_y_q4};
    [col_Ja_4, T_4_0] = transformacoesCombinadas(T_3_0,transformacoesPuras_4_3);
    P_4_0 = T_4_0(1:3, 4);
    
    %% {5} Ferramenta:
    D_5_4_P5 = TranslacaoPura(P_5);
    transformacoesPuras_5_4 = {D_5_4_P5};
    [col_Ja_5, T_5_0] = transformacoesCombinadas(T_4_0,transformacoesPuras_5_4);
    P_5_0 = T_5_0(1:3, 4);
    
    posicoes = P_5_0
    
    %% Velocidades com os jacobianos ja calculados
    velocidades = [- dq1*(L2*sin(q1 + q2) + L1*sin(q1)) - L2*dq2*sin(q1 + q2); dq3; - dq1*(L2*cos(q1 + q2) + L1*cos(q1)) - L2*dq2*cos(q1 + q2)];
    
    %% Aceleracoes com as derivadas temporais dos Jacobianos lineares ja calculadas

    aceleracoes = [- d2q1*(L2*sin(q1 + q2) + L1*sin(q1)) - dq2*(L2*dq1*cos(q1 + q2) + L2*dq2*cos(q1 + q2)) - dq1*(dq1*(L2*cos(q1 + q2) + L1*cos(q1)) ...
        + L2*dq2*cos(q1 + q2)) - L2*d2q2*sin(q1 + q2); d2q3; dq2*(L2*dq1*sin(q1 + q2) + L2*dq2*sin(q1 + q2)) - d2q1*(L2*cos(q1 + q2) + L1*cos(q1)) ...
        + dq1*(dq1*(L2*sin(q1 + q2) + L1*sin(q1)) + L2*dq2*sin(q1 + q2)) - L2*d2q2*cos(q1 + q2)];

end

== matlab function simulacao_manipulador_scara_Anne/MATLAB Function2 ==
  data: d2q output; Tc input; M input; G input; H input; D input
function d2q   = planta(Tc, M, G, H, D) % a planta devolve a aceleração simulada
d2q = M\(Tc-H-G-D);

== matlab function simulacao_manipulador_scara_Anne/matriz_massa_M ==
  data: q2 input; M output; q4 input
function M = matriz_massa_M(q2,q4)
%#codegen

%    This function was generated by the Symbolic Math Toolbox version 24.2.
%    25-Sep-2024 18:08:50

% q2 = complex(q2);  % if required to enforce complex operations
% q4 = complex(q4);  % if required to enforce complex operations
t2 = cos(q2);
t3 = cos(q4);
t4 = sin(q2);
t5 = q2+q4;
t6 = cos(t5);
t7 = t3.*1.908522e-6;
t8 = t3.*3.817044e-6;
t13 = t4.*1.5345288e-6;
t15 = t2.*1.399767764724e-1;
t9 = t6.*3.036285e-6;
t10 = -t8;
t11 = -t7;
t14 = -t13;
t12 = -t9;
t16 = t11+9.001821771e-6;
t17 = t12+t16;
t18 = t10+t12+t14+t15+6.725829196394252e-2;
et1 = t2.*2.799535529448e-1-t4.*3.0690576e-6-t6.*6.07257e-6+t10;
et2 = 5.438445764595695e-1;
mt1 = [et1+et2,t18,0.0,t17,t18,t10+6.725829196394252e-2,0.0,t16,0.0,0.0,4.4243e-2,0.0,t17,t16,0.0];
mt2 = [9.001821771e-6];
M = reshape([mt1,mt2],4,4);
end

== matlab function simulacao_manipulador_scara_Anne/gravidade_G ==
  data: G output
function G = gravidade_G
%#codegen

%    This function was generated by the Symbolic Math Toolbox version 24.2.
%    25-Sep-2024 18:08:51

G = [0.0;0.0;4.3402383e-1;0.0];
end

== matlab function simulacao_manipulador_scara_Anne/centrifuga_coriolis_H ==
  data: dq1 input; H output; dq2 input; dq4 input; q2 input; q4 input
function H = centrifuga_coriolis_H(dq1,dq2,dq4,q2,q4)
%#codegen

%    This function was generated by the Symbolic Math Toolbox version 24.2.
%    25-Sep-2024 18:08:51

% dq1 = complex(dq1);  % if required to enforce complex operations
% dq2 = complex(dq2);  % if required to enforce complex operations
% dq4 = complex(dq4);  % if required to enforce complex operations
% q2 = complex(q2);  % if required to enforce complex operations
% q4 = complex(q4);  % if required to enforce complex operations
t2 = cos(q2);
t3 = sin(q2);
t4 = sin(q4);
t5 = q2+q4;
t6 = dq1.^2;
t7 = dq2.^2;
t8 = dq4.^2;
t9 = sin(t5);
t10 = dq1.*dq4.*t4.*3.817044e-6;
t11 = dq2.*dq4.*t4.*3.817044e-6;
t12 = t4.*t8.*1.908522e-6;
t13 = t6.*t9.*3.036285e-6;
t14 = -t13;
et1 = t10+t11+t12-t2.*t7.*1.5345288e-6-t3.*t7.*1.399767764724e-1+t7.*t9.*3.036285e-6;
et2 = t8.*t9.*3.036285e-6-dq1.*dq2.*t2.*3.0690576e-6-dq1.*dq2.*t3.*2.799535529448e-1;
et3 = dq1.*dq2.*t9.*6.07257e-6+dq1.*dq4.*t9.*6.07257e-6+dq2.*dq4.*t9.*6.07257e-6;
mt1 = [et1+et2+et3;t10+t11+t12+t14+t2.*t6.*1.5345288e-6+t3.*t6.*1.399767764724e-1;0.0];
mt2 = [t14-t4.*t6.*1.908522e-6-t4.*t7.*1.908522e-6-dq1.*dq2.*t4.*3.817044e-6];
H = [mt1;mt2];
end
